simulink model "Model_simulink_dyskretny_no_torque"  (R2017a)
settings: Solver=ode45  StartTime=0.0  StopTime=Tend  FixedStep=Tp  RelTol=1e-3
undefined symbols (not defined in the file): In, J, K1, K2, K3, K4, Kp, Kt, Lambda, psi, Rt, T, Tp, Un, Uz0, wn, Y
settings Model: Creator=user  LastModifiedBy=a
settings DataIOCC: LimitDataPoints=on  SaveFormat=Array  SignalLoggingSaveFormat=ModelDataLogs
settings OptimizationCC: BlockReduction=off  BooleanDataType=off  ExpressionDepthLimit=2147483647  LifeSpan=inf
settings DebuggingCC: SaveWithParameterizedLinksMsg=none  UnderspecifiedInitializationDetection=Classic  MergeDetectMultiDrivingBlocksExec=none  SignalResolutionControl=TryResolveAllWithWarning  MultiTaskDSMMsg=warning  MultiTaskCondExecSysMsg=none  StateNameClashWarn=warning  SFUnexpectedBacktrackingDiag=warning  SFNoUnconditionalDefaultTransitionDiag=warning  SFExecutionAtInitializationDiag=none
settings HardwareCC: ProdBitPerPointer=32  ProdBitPerSizeT=32  ProdBitPerPtrDiffT=32  ProdLargestAtomicFloat=None  ProdIntDivRoundTo=Undefined  ProdEndianess=Unspecified  ProdWordSize=32  ProdHWDeviceType=32-bit Generic  TargetUnknown=on
settings ModelReferenceCC: PropagateSignalLabelsOutOfModel=off
settings GRTTargetCC: TargetLangStandard=C89/C90 (ANSI)  GeneratePreprocessorConditionals=Disable all
settings ConfigComp: CovMetricSettings=dw  CovHtmlReporting=on  CovSaveCumulativeToWorkspaceVar=on  CovSaveSingleToWorkspaceVar=on  CovExternalEMLEnable=off

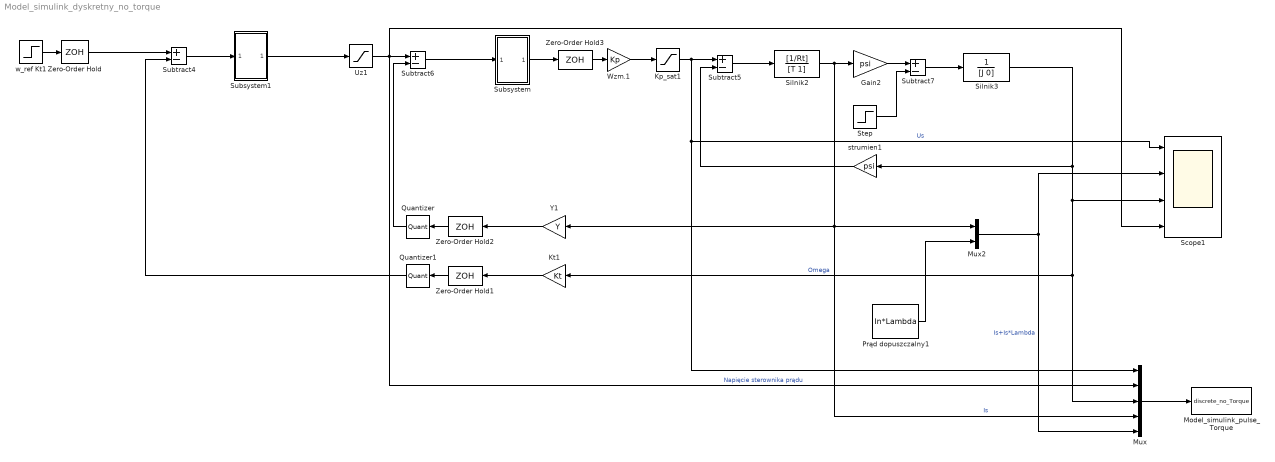
== system Model_simulink_dyskretny_no_torque ==
  Gain2 : Gain  Gain=psi
  Kp_sat1 : Saturate  UpperLimit=1.5*Un  LowerLimit=-1.5*Un
  Kt1 : Gain  Gain=Kt
  Model_simulink_pulse_Torque : ToWorkspace  VariableName=discrete_no_Torque  SaveFormat=Structure With Time  SampleTime=Tp
  Mux : Mux  Inputs=5
  Mux2 : Mux  Inputs=2
  Prąd dopuszczalny1 : Constant  Value=In*Lambda
  Quantizer : Quantizer  QuantizationInterval=Q
  Quantizer1 : Quantizer  QuantizationInterval=Q
  Scope1 : Scope  NumInputPorts=4
  Silnik2 : TransferFcn  Numerator=[1/Rt]  Denominator=[T 1]
  Silnik3 : TransferFcn  Numerator=1  Denominator=[J 0]
  Step : Step  After=0  SampleTime=0
  Subsystem : Subsystem
  Subsystem1 : Subsystem
  Subtract{4..7} (4 alike) : Sum  Inputs=+-
  Uz1 : Saturate  UpperLimit=Uz0  LowerLimit=-Uz0
  Wzm.1 : Gain  Gain=Kp
  Y1 : Gain  Gain=Y
  Zero-Order Hold{,1..3} (4 alike) : ZeroOrderHold  SampleTime=Tp
  strumien1 : Gain  Gain=psi
  w_ref Kt1 : Step  Time=0  After=wn*Kt  SampleTime=0
  wires:
  Wzm.1/1 -> Kp_sat1/1
  Subtract5/1 -> Silnik2/1
  Silnik2/1 -> Mux/4, Y1/1, Mux2/1, Gain2/1  "Is"
  Gain2/1 -> Subtract7/1
  Subtract7/1 -> Silnik3/1
  strumien1/1 -> Subtract5/2
  Kp_sat1/1 -> Mux/1, Scope1/1, Subtract5/1  "Us"
  Y1/1 -> Zero-Order Hold2/1
  Mux2/1 -> Mux/5, Scope1/2  "Is+Is*Lambda"
  Prąd dopuszczalny1/1 -> Mux2/2
  Uz1/1 -> Mux/2, Scope1/4, Subtract6/1  "Napięcie sterownika prądu"
  Silnik3/1 -> Mux/3, Kt1/1, Scope1/3, strumien1/1  "Omega"
  Kt1/1 -> Zero-Order Hold1/1
  Step/1 -> Subtract7/2
  Mux/1 -> Model_simulink_pulse_Torque/1
  Subtract6/1 -> Subsystem/1(In1)
  Subsystem1/1(Out1) -> Uz1/1
  Subtract4/1 -> Subsystem1/1(In1)
  Zero-Order Hold2/1 -> Quantizer/1
  Zero-Order Hold1/1 -> Quantizer1/1
  Quantizer/1 -> Subtract6/2
  Quantizer1/1 -> Subtract4/2
  Zero-Order Hold/1 -> Subtract4/1
  Zero-Order Hold3/1 -> Wzm.1/1
  Subsystem/1(Out1) -> Zero-Order Hold3/1
  w_ref Kt1/1 -> Zero-Order Hold/1

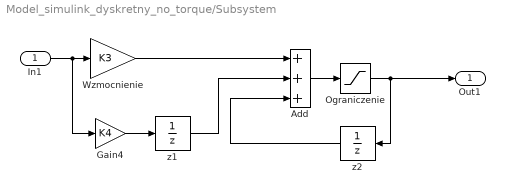
== system Model_simulink_dyskretny_no_torque/Subsystem ==
  In1 : Inport
  Add : Sum  Inputs=+++
  Gain4 : Gain  Gain=K4  SampleTime=Tp
  Ograniczenie : Saturate  UpperLimit=10  LowerLimit=-10  SampleTime=Tp
  Wzmocnienie : Gain  Gain=K3  SampleTime=Tp
  z1 : UnitDelay  SampleTime=Tp
  z2 : UnitDelay  SampleTime=Tp
  Out1 : Outport
  wires:
  In1/1 -> Gain4/1, Wzmocnienie/1
  Wzmocnienie/1 -> Add/1
  Gain4/1 -> z1/1
  z1/1 -> Add/2
  Add/1 -> Ograniczenie/1
  Ograniczenie/1 -> Out1/1, z2/1
  z2/1 -> Add/3

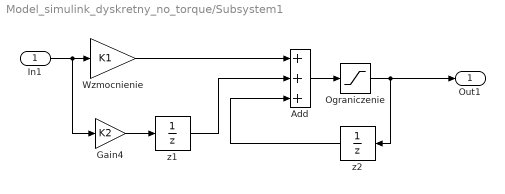
== system Model_simulink_dyskretny_no_torque/Subsystem1 ==
  In1 : Inport
  Add : Sum  Inputs=+++
  Gain4 : Gain  Gain=K2  SampleTime=Tp
  Ograniczenie : Saturate  UpperLimit=10  LowerLimit=-10
  Wzmocnienie : Gain  Gain=K1  SampleTime=Tp
  z1 : UnitDelay  SampleTime=Tp
  z2 : UnitDelay  SampleTime=Tp
  Out1 : Outport
  wires:
  In1/1 -> Gain4/1, Wzmocnienie/1
  Wzmocnienie/1 -> Add/1
  Gain4/1 -> z1/1
  z1/1 -> Add/2
  Add/1 -> Ograniczenie/1
  Ograniczenie/1 -> Out1/1, z2/1
  z2/1 -> Add/3
